simulink model "Plant"  (R2020a)
settings: Solver=VariableStepAuto  StartTime=0.0  StopTime=120  RelTol=1e-3
undefined symbols (not defined in the file): b, m
settings Model: DataDictionary=Week2_Problem3.sldd  Creator=sreeram  LastModifiedBy=sreeram
settings DataIOCC: SaveOutput=off  SaveTime=off

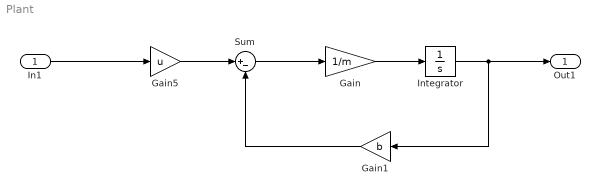
== system Plant ==
  In1 : Inport  OutDataTypeStr=double  PortDimensions=1  SampleTime=0
  Gain : Gain  Gain=1/m
  Gain1 : Gain  Gain=b
  Gain5 : Gain  Gain=u
  Integrator : Integrator
  Sum : Sum  Inputs=|+-
  Out1 : Outport  OutDataTypeStr=double  PortDimensions=1  SampleTime=0
  wires:
  Gain/1 -> Integrator/1
  Sum/1 -> Gain/1
  Integrator/1 -> Gain1/1, Out1/1
  Gain5/1 -> Sum/1
  Gain1/1 -> Sum/2
  In1/1 -> Gain5/1
